simulink model "untitled"  (R2012b)
settings: Solver=ode3  StartTime=0.0  StopTime=1  FixedStep=1e-4  RelTol=1e-3
libraries: simulink x3, powerlib_extras x2
settings Model: Creator=h3now  LastModifiedBy=h3now

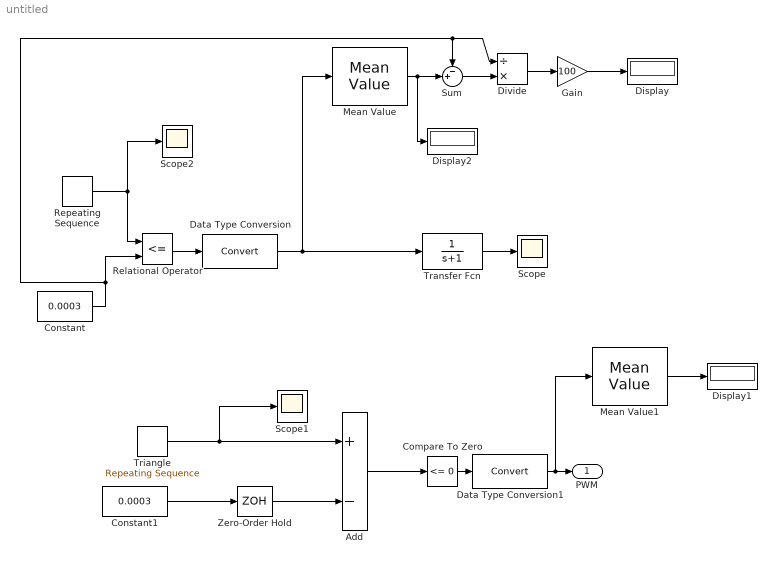
== system untitled ==
  Add : Sum  Inputs=+-  SampleTime=1/10000
  Compare To Zero : simulink/Logic and Bit Operations/Compare To Zero  relop=<=  OutDataTypeStr=uint8
  Constant : Constant  Value=0.0003
  Constant1 : Constant  Value=0.0003
  Data Type Conversion : DataTypeConversion
  Data Type Conversion1 : DataTypeConversion
  Display : Display
  Display1 : Display
  Display2 : Display
  Divide : Product  Inputs=/*
  Gain : Gain  Gain=100
  Mean Value : powerlib_extras/Measurements/Mean Value  Period=1
  Mean Value1 : powerlib_extras/Measurements/Mean Value  Period=1
  Relational Operator : RelationalOperator  Operator=<=  OutDataTypeStr=boolean
  Repeating Sequence : simulink/Sources/Repeating Sequence  rep_seq_t=[0 1/100]  rep_seq_y=[0 1]
  Scope : Scope
      settings: YMin=0.3  YMax=2.6
  Scope1 : Scope
      settings: SaveName=ScopeData3
  Scope2 : Scope
      settings: YMin=0.294  YMax=0.301  SaveName=ScopeData2
  Sum : Sum  Inputs=-+|
  Transfer Fcn : TransferFcn  Denominator=[1 1]
  Triangle : simulink/Sources/Repeating Sequence  rep_seq_t=[0 1/100/4 3/100/4 1/100]  rep_seq_y=[0.5 0 1 0.5]
  Zero-Order Hold : ZeroOrderHold  SampleTime=1/10000
  PWM : Outport
  wires:
  Constant/1 -> Sum/1, Divide/1, Relational Operator/2
  Repeating Sequence/1 -> Relational Operator/1, Scope2/1
  Relational Operator/1 -> Data Type Conversion/1
  Transfer Fcn/1 -> Scope/1
  Data Type Conversion/1 -> Mean Value/1, Transfer Fcn/1
  Mean Value/1 -> Display2/1, Sum/2
  Sum/1 -> Divide/2
  Divide/1 -> Gain/1
  Gain/1 -> Display/1
  Triangle/1 -> Scope1/1, Add/1
  Constant1/1 -> Zero-Order Hold/1
  Add/1 -> Compare To Zero/1
  Zero-Order Hold/1 -> Add/2
  Mean Value1/1 -> Display1/1
  Compare To Zero/1 -> Data Type Conversion1/1
  Data Type Conversion1/1 -> Mean Value1/1, PWM/1
